simulink model "simcape_real_time_V3"  (R2022b)
settings: Solver=FixedStepAuto  StartTime=0.0  StopTime=100  FixedStep=0.002  RelTol=1e-3
undefined symbols (not defined in the file): drone_leg, K_LQR_GOC, pitch_init, roll_init, v_pitch_init, v_roll_init, v_x_init, v_y_init, v_yaw_init, v_z_init, X, x_init, Y, y_init, yaw_init, Z, z_init
libraries: sm_lib x70, nesl_utility x11, simulink x6
(part 3 of 4)

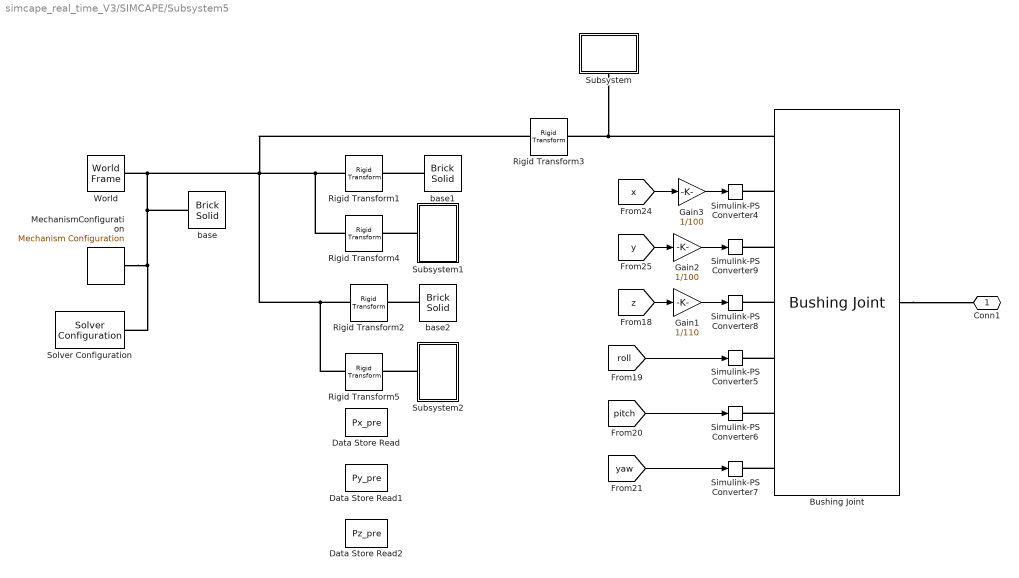
== system simcape_real_time_V3/SIMCAPE/Subsystem5 ==
  Bushing Joint : sm_lib/Joints/Bushing Joint  JointMode=Normal  SenseConstraintForce=off  SenseConstraintForceX=off  SenseConstraintForceY=off  SenseConstraintForceZ=off  SenseConstraintTorque=off  SenseConstraintTorqueX=off  SenseConstraintTorqueY=off  SenseConstraintTorqueZ=off  SenseTotalForce=off  SenseTotalForceX=off  SenseTotalForceY=off  SenseTotalForceZ=off  SenseTotalTorque=off  SenseTotalTorqueX=off  SenseTotalTorqueY=off  SenseTotalTorqueZ=off  CompositeWrenchDir=FollowerOnBase  CompositeWrenchFrame=BaseFrame  PxEquilibriumPosition=0  PxEquilibriumPositionUnits=m  PxSpringStiffness=0  PxSpringStiffnessUnits=N/m  PxDampingCoefficient=0  PxDampingCoefficientUnits=N/(m/s)  PxTorqueActuationMode=ComputedTorque  PxMotionActuationMode=InputMotion  PxSensePosition=off  PxSenseVelocity=off  PxSenseAcceleration=off  PxSenseTorqueForce=off  PxSenseLowerLimitTorqueForce=off  PxSenseUpperLimitTorqueForce=off  PxLowerLimitSpecify=off  PxLowerLimitBound=-1  PxLowerLimitBoundUnits=m  PxLowerLimitStiffness=1e6  PxLowerLimitStiffnessUnits=N/m  PxLowerLimitDamping=1e3  PxLowerLimitDampingUnits=N/(m/s)  PxLowerLimitTransitionRegionWidth=1e-4  PxLowerLimitTransitionRegionWidthUnits=m  PxUpperLimitSpecify=off  PxUpperLimitBound=1  PxUpperLimitBoundUnits=m  PxUpperLimitStiffness=1e6  PxUpperLimitStiffnessUnits=N/m  PxUpperLimitDamping=1e3  PxUpperLimitDampingUnits=N/(m/s)  PxUpperLimitTransitionRegionWidth=1e-4  PxUpperLimitTransitionRegionWidthUnits=m  PxPositionTargetSpecify=off  PxPositionTargetPriority=High  PxPositionTargetValue=0  PxPositionTargetValueUnits=m  PxVelocityTargetSpecify=off  PxVelocityTargetPriority=High  PxVelocityTargetValue=0  PxVelocityTargetValueUnits=m/s  PyEquilibriumPosition=0  PyEquilibriumPositionUnits=m  PySpringStiffness=0  PySpringStiffnessUnits=N/m  PyDampingCoefficient=0  PyDampingCoefficientUnits=N/(m/s)  PyTorqueActuationMode=ComputedTorque  PyMotionActuationMode=InputMotion  PySensePosition=off  PySenseVelocity=off  PySenseAcceleration=off  PySenseTorqueForce=off  PySenseLowerLimitTorqueForce=off  PySenseUpperLimitTorqueForce=off  PyLowerLimitSpecify=off  PyLowerLimitBound=-1  PyLowerLimitBoundUnits=m  PyLowerLimitStiffness=1e6  PyLowerLimitStiffnessUnits=N/m  PyLowerLimitDamping=1e3  PyLowerLimitDampingUnits=N/(m/s)  PyLowerLimitTransitionRegionWidth=1e-4  PyLowerLimitTransitionRegionWidthUnits=m  PyUpperLimitSpecify=off  PyUpperLimitBound=1  PyUpperLimitBoundUnits=m  PyUpperLimitStiffness=1e6  PyUpperLimitStiffnessUnits=N/m  PyUpperLimitDamping=1e3  PyUpperLimitDampingUnits=N/(m/s)  PyUpperLimitTransitionRegionWidth=1e-4  PyUpperLimitTransitionRegionWidthUnits=m  PyPositionTargetSpecify=off  PyPositionTargetPriority=High  PyPositionTargetValue=0  PyPositionTargetValueUnits=m  PyVelocityTargetSpecify=off  PyVelocityTargetPriority=High  PyVelocityTargetValue=0  PyVelocityTargetValueUnits=m/s  PzEquilibriumPosition=0  PzEquilibriumPositionUnits=m  PzSpringStiffness=0  PzSpringStiffnessUnits=N/m  PzDampingCoefficient=0  PzDampingCoefficientUnits=N/(m/s)  PzTorqueActuationMode=ComputedTorque  PzMotionActuationMode=InputMotion  PzSensePosition=off  PzSenseVelocity=off  PzSenseAcceleration=off  PzSenseTorqueForce=off  PzSenseLowerLimitTorqueForce=off  PzSenseUpperLimitTorqueForce=off  PzLowerLimitSpecify=off  PzLowerLimitBound=-1  PzLowerLimitBoundUnits=m  PzLowerLimitStiffness=1e6  PzLowerLimitStiffnessUnits=N/m  PzLowerLimitDamping=1e3  PzLowerLimitDampingUnits=N/(m/s)  PzLowerLimitTransitionRegionWidth=1e-4  PzLowerLimitTransitionRegionWidthUnits=m  PzUpperLimitSpecify=off  PzUpperLimitBound=1  PzUpperLimitBoundUnits=m  PzUpperLimitStiffness=1e6  PzUpperLimitStiffnessUnits=N/m  PzUpperLimitDamping=1e3  PzUpperLimitDampingUnits=N/(m/s)  PzUpperLimitTransitionRegionWidth=1e-4  PzUpperLimitTransitionRegionWidthUnits=m  PzPositionTargetSpecify=off  PzPositionTargetPriority=High  PzPositionTargetValue=0  PzPositionTargetValueUnits=m  PzVelocityTargetSpecify=off  PzVelocityTargetPriority=High  PzVelocityTargetValue=0  PzVelocityTargetValueUnits=m/s  RxEquilibriumPosition=0  RxEquilibriumPositionUnits=deg  RxSpringStiffness=0  RxSpringStiffnessUnits=N*m/deg  RxDampingCoefficient=0  RxDampingCoefficientUnits=N*m/(deg/s)  RxTorqueActuationMode=ComputedTorque  RxMotionActuationMode=InputMotion  RxSensePosition=off  RxSenseVelocity=off  RxSenseAcceleration=off  RxSenseTorqueForce=off  RxSenseLowerLimitTorqueForce=off  RxSenseUpperLimitTorqueForce=off  RxLowerLimitSpecify=off  RxLowerLimitBound=-90  RxLowerLimitBoundUnits=deg  RxLowerLimitStiffness=1e4  RxLowerLimitStiffnessUnits=N*m/deg  RxLowerLimitDamping=10  RxLowerLimitDampingUnits=N*m/(deg/s)  RxLowerLimitTransitionRegionWidth=0.1  RxLowerLimitTransitionRegionWidthUnits=deg  RxUpperLimitSpecify=off  RxUpperLimitBound=90  RxUpperLimitBoundUnits=deg  RxUpperLimitStiffness=1e4  RxUpperLimitStiffnessUnits=N*m/deg  RxUpperLimitDamping=10  RxUpperLimitDampingUnits=N*m/(deg/s)  RxUpperLimitTransitionRegionWidth=0.1  RxUpperLimitTransitionRegionWidthUnits=deg  RxPositionTargetSpecify=off  RxPositionTargetPriority=High  RxPositionTargetValue=0  RxPositionTargetValueUnits=deg  RxVelocityTargetSpecify=off  RxVelocityTargetPriority=High  RxVelocityTargetValue=0  RxVelocityTargetValueUnits=deg/s  RyEquilibriumPosition=0  RyEquilibriumPositionUnits=deg  RySpringStiffness=0  RySpringStiffnessUnits=N*m/deg  RyDampingCoefficient=0  RyDampingCoefficientUnits=N*m/(deg/s)  RyTorqueActuationMode=ComputedTorque  RyMotionActuationMode=InputMotion  RySensePosition=off  RySenseVelocity=off  RySenseAcceleration=off  RySenseTorqueForce=off  RySenseLowerLimitTorqueForce=off  RySenseUpperLimitTorqueForce=off  RyLowerLimitSpecify=off  RyLowerLimitBound=-90  RyLowerLimitBoundUnits=deg  RyLowerLimitStiffness=1e4  RyLowerLimitStiffnessUnits=N*m/deg  RyLowerLimitDamping=10  RyLowerLimitDampingUnits=N*m/(deg/s)  RyLowerLimitTransitionRegionWidth=0.1  RyLowerLimitTransitionRegionWidthUnits=deg  RyUpperLimitSpecify=off  RyUpperLimitBound=90  RyUpperLimitBoundUnits=deg  RyUpperLimitStiffness=1e4  RyUpperLimitStiffnessUnits=N*m/deg  RyUpperLimitDamping=10  RyUpperLimitDampingUnits=N*m/(deg/s)  RyUpperLimitTransitionRegionWidth=0.1  RyUpperLimitTransitionRegionWidthUnits=deg  RyPositionTargetSpecify=off  RyPositionTargetPriority=High  RyPositionTargetValue=0  RyPositionTargetValueUnits=deg  RyVelocityTargetSpecify=off  RyVelocityTargetPriority=High  RyVelocityTargetValue=0  RyVelocityTargetValueUnits=deg/s  RzEquilibriumPosition=0  RzEquilibriumPositionUnits=deg  RzSpringStiffness=0  RzSpringStiffnessUnits=N*m/deg  RzDampingCoefficient=0  RzDampingCoefficientUnits=N*m/(deg/s)  RzTorqueActuationMode=ComputedTorque  RzMotionActuationMode=InputMotion  RzSensePosition=off  RzSenseVelocity=off  RzSenseAcceleration=off  RzSenseTorqueForce=off  RzSenseLowerLimitTorqueForce=off  RzSenseUpperLimitTorqueForce=off  RzLowerLimitSpecify=off  RzLowerLimitBound=-90  RzLowerLimitBoundUnits=deg  RzLowerLimitStiffness=1e4  RzLowerLimitStiffnessUnits=N*m/deg  RzLowerLimitDamping=10  RzLowerLimitDampingUnits=N*m/(deg/s)  RzLowerLimitTransitionRegionWidth=0.1  RzLowerLimitTransitionRegionWidthUnits=deg  RzUpperLimitSpecify=off  RzUpperLimitBound=90  RzUpperLimitBoundUnits=deg  RzUpperLimitStiffness=1e4  RzUpperLimitStiffnessUnits=N*m/deg  RzUpperLimitDamping=10  RzUpperLimitDampingUnits=N*m/(deg/s)  RzUpperLimitTransitionRegionWidth=0.1  RzUpperLimitTransitionRegionWidthUnits=deg  RzPositionTargetSpecify=off  RzPositionTargetPriority=High  RzPositionTargetValue=0  RzPositionTargetValueUnits=deg  RzVelocityTargetSpecify=off  RzVelocityTargetPriority=High  RzVelocityTargetValue=0  RzVelocityTargetValueUnits=deg/s
  Data Store Read : DataStoreRead  DataStoreName=Px_pre  IndexOptions=Index vector (dialog)  Indices=1  OutputSizes=1
  Data Store Read1 : DataStoreRead  DataStoreName=Py_pre  IndexOptions=Index vector (dialog)  Indices=1  OutputSizes=1
  Data Store Read2 : DataStoreRead  DataStoreName=Pz_pre  IndexOptions=Index vector (dialog)  Indices=1  OutputSizes=1
  Gain1 : Gain  Gain=1/110
  Gain2 : Gain  Gain=1/100
  Gain3 : Gain  Gain=1/100
  MechanismConfiguration : sm_lib/Utilities/Mechanism Configuration  UniformGravity=Constant  GravityVector=[0 -9.81 0]  GravityUnits=m/s^2  LinearizationDelta=0.002  JointModeTransitionNonlinearIterations=2
  Rigid Transform1 : sm_lib/Frames and Transforms/Rigid Transform  TranslationMethod=Cartesian  TranslationStandardOffset=45  TranslationLengthUnit=cm  TranslationStandardAxis=+Y  TranslationCartesianOffset=[0 300 -50]  TranslationROffset=0  TranslationROffsetUnits=m  TranslationZOffset=0  TranslationZOffsetUnits=m  TranslationThetaOffset=0  TranslationThetaOffsetUnits=deg  RotationMethod=StandardAxis  RotationAngleUnits=deg  RotationStandardAxis=+Z  RotationAngle=90  RotationArbitraryAxis=[0 0 1]  FollAlignAxisA=+X  BaseAlignAxisA=+Y  FollAlignAxisB=+Y  BaseAlignAxisB=+Z  RotationSequenceAxes=FollowerAxes  RotationSequence=XYX  RotationSequenceAngles=[0 0 0]  RotationSequenceAnglesUnits=deg  RotationMatrix=[1 0 0; 0 1 0; 0 0 1]  Quaternion=[1 0 0 0]
  Rigid Transform2 : sm_lib/Frames and Transforms/Rigid Transform  TranslationMethod=Cartesian  TranslationStandardOffset=45  TranslationLengthUnit=cm  TranslationStandardAxis=+Y  TranslationCartesianOffset=[300 0 -100]  TranslationROffset=0  TranslationROffsetUnits=m  TranslationZOffset=0  TranslationZOffsetUnits=m  TranslationThetaOffset=0  TranslationThetaOffsetUnits=deg  RotationMethod=StandardAxis  RotationAngleUnits=deg  RotationStandardAxis=+Z  RotationAngle=90  RotationArbitraryAxis=[0 0 1]  FollAlignAxisA=+X  BaseAlignAxisA=+Y  FollAlignAxisB=+Y  BaseAlignAxisB=+Z  RotationSequenceAxes=FollowerAxes  RotationSequence=XYX  RotationSequenceAngles=[0 0 0]  RotationSequenceAnglesUnits=deg  RotationMatrix=[1 0 0; 0 1 0; 0 0 1]  Quaternion=[1 0 0 0]
  Rigid Transform3 : sm_lib/Frames and Transforms/Rigid Transform  TranslationMethod=Cartesian  TranslationStandardOffset=45  TranslationLengthUnit=cm  TranslationStandardAxis=+Y  TranslationCartesianOffset=[0 -0 -30]  TranslationROffset=0  TranslationROffsetUnits=m  TranslationZOffset=0  TranslationZOffsetUnits=m  TranslationThetaOffset=0  TranslationThetaOffsetUnits=deg  RotationMethod=StandardAxis  RotationAngleUnits=deg  RotationStandardAxis=+Z  RotationAngle=90  RotationArbitraryAxis=[0 0 1]  FollAlignAxisA=+X  BaseAlignAxisA=+Y  FollAlignAxisB=+Y  BaseAlignAxisB=+Z  RotationSequenceAxes=FollowerAxes  RotationSequence=XYX  RotationSequenceAngles=[0 0 0]  RotationSequenceAnglesUnits=deg  RotationMatrix=[1 0 0; 0 1 0; 0 0 1]  Quaternion=[1 0 0 0]
  Rigid Transform4 : sm_lib/Frames and Transforms/Rigid Transform  TranslationMethod=Cartesian  TranslationStandardOffset=45  TranslationLengthUnit=cm  TranslationStandardAxis=+Y  TranslationCartesianOffset=[0 300 -80]  TranslationROffset=0  TranslationROffsetUnits=m  TranslationZOffset=0  TranslationZOffsetUnits=m  TranslationThetaOffset=0  TranslationThetaOffsetUnits=deg  RotationMethod=StandardAxis  RotationAngleUnits=deg  RotationStandardAxis=+Z  RotationAngle=90  RotationArbitraryAxis=[0 0 1]  FollAlignAxisA=+X  BaseAlignAxisA=+Y  FollAlignAxisB=+Y  BaseAlignAxisB=+Z  RotationSequenceAxes=FollowerAxes  RotationSequence=XYX  RotationSequenceAngles=[0 0 0]  RotationSequenceAnglesUnits=deg  RotationMatrix=[1 0 0; 0 1 0; 0 0 1]  Quaternion=[1 0 0 0]
  Rigid Transform5 : sm_lib/Frames and Transforms/Rigid Transform  TranslationMethod=Cartesian  TranslationStandardOffset=45  TranslationLengthUnit=cm  TranslationStandardAxis=+Y  TranslationCartesianOffset=[300 0 -130]  TranslationROffset=0  TranslationROffsetUnits=m  TranslationZOffset=0  TranslationZOffsetUnits=m  TranslationThetaOffset=0  TranslationThetaOffsetUnits=deg  RotationMethod=StandardAxis  RotationAngleUnits=deg  RotationStandardAxis=+Z  RotationAngle=90  RotationArbitraryAxis=[0 0 1]  FollAlignAxisA=+X  BaseAlignAxisA=+Y  FollAlignAxisB=+Y  BaseAlignAxisB=+Z  RotationSequenceAxes=FollowerAxes  RotationSequence=XYX  RotationSequenceAngles=[0 0 0]  RotationSequenceAnglesUnits=deg  RotationMatrix=[1 0 0; 0 1 0; 0 0 1]  Quaternion=[1 0 0 0]
  Simulink-PS Converter{4..9} (6 alike) : nesl_utility/Simulink-PS Converter  PhysicalDomain=network_engine_domain  SubClassName=ps_input  LeftPortType=input  RightPortType=output  PseudoPeriodic=off  Frequencies=[]  NoiseDistribution=none  NoiseParameters=[]  Unit=1  AffineConversion=off  FilteringAndDerivatives=filter  SimscapeFilterOrder=2  InputFilterTimeConstant=0.002  UdotUserProvided=0
  Solver Configuration : nesl_utility/Solver Configuration  PhysicalDomain=network_engine_domain  SubClassName=solver  LeftPortType=input  RightPortType=generic  Tones=[]  Harmonics=[]  SimulateNoise=off  Profile=off  UseLocalSampling=off  EnableSwitchedLinearOptims=on  FrequencyDomain=off  UseCCode=off  RelTol=0.001  AbsTol=1e-06  MinStep=1e-09  ToWorkspace=off  RevertToSquareIcSolve=off  NumHomotopyIterations=100  PhasorMode=off  PhasorModeNumHarmonics=1  ConsistencySolver=NEWTON_FTOL  IndexReductionMethod=DerivativeReplacement  DoDC=off  ResidualTolerance=1e-09  ConsistencyTolSource=GLOBAL  ConsistencyAbsTol=0.001  ConsistencyRelTol=0.001  ConsistencyTolFactor=0.001  UseLocalSolver=off  LocalSolverChoice=NE_BACKWARD_EULER_ADVANCER  ResolveIndetEquations=on  FunctionEvalNumThread=1  LocalSolverSampleTime=0.001  DoFixedCost=off  MaxNonlinIter=3  MaxModeIter=2  ComputeImpulses=off  ImpulseIterations=2  LinearAlgebra=Sparse  LinearAlgebraNumThread=0  EquationFormulation=NE_TIME_EF  DelaysMemoryBudget=1024  AutomaticFiltering=on  FilteringTimeConstant=0.001  PartitionStorageMethod=AS_NEEDED  PartitionMemoryBudget=1024  PartitionMethod=FAST
  Subsystem : Subsystem
  Subsystem1 : Subsystem
  Subsystem2 : Subsystem
  World : sm_lib/Frames and Transforms/World Frame
  base : sm_lib/Body Elements/Brick Solid  GraphicAmbientColor=[0.15 0.9 0.15 1.0]  BasedOnType=Density  BrickDimensions=[300 300 50]  BrickDimensionUnits=cm  CenterOfMass=[0 0 0]  CenterOfMassUnits=m  GraphicDiffuseColor=[0.0 0.8 0.0]  Density=1000  DensityUnits=kg/(m^3)  DoExposeReferenceFrame=on  GraphicEmissiveColor=[0.0 0.0 0.0 1.0]  ExportEntireGeometry=off  SerializedFrames=<Frames/>  MarkerShape=Sphere  MarkerSize=10  GraphicType=FromGeometry  InertiaType=CalculateFromGeometry  Mass=1  MassUnits=kg  MomentsOfInertia=[1 1 1]  MomentsOfInertiaUnits=kg*m^2  GraphicOpacity=1.0  ProductsOfInertia=[0 0 0]  ProductsOfInertiaUnits=kg*m^2  GraphicShininess=75  GraphicSpecularColor=[0.5 0.5 0.5 1.0]  GraphicVisPropType=SimpleVisualProperties
  base1 : sm_lib/Body Elements/Brick Solid  GraphicAmbientColor=[0.15 0.9 0.15 1.0]  BasedOnType=Density  BrickDimensions=[300 300 50]  BrickDimensionUnits=cm  CenterOfMass=[0 0 0]  CenterOfMassUnits=m  GraphicDiffuseColor=[0.4 1.0 1.0]  Density=1000  DensityUnits=kg/(m^3)  DoExposeReferenceFrame=on  GraphicEmissiveColor=[0.0 0.0 0.0 1.0]  ExportEntireGeometry=off  SerializedFrames=<Frames/>  MarkerShape=Sphere  MarkerSize=10  GraphicType=FromGeometry  InertiaType=CalculateFromGeometry  Mass=1  MassUnits=kg  MomentsOfInertia=[1 1 1]  MomentsOfInertiaUnits=kg*m^2  GraphicOpacity=1.0  ProductsOfInertia=[0 0 0]  ProductsOfInertiaUnits=kg*m^2  GraphicShininess=75  GraphicSpecularColor=[0.5 0.5 0.5 1.0]  GraphicVisPropType=SimpleVisualProperties
  base2 : sm_lib/Body Elements/Brick Solid  GraphicAmbientColor=[0.15 0.9 0.15 1.0]  BasedOnType=Density  BrickDimensions=[300 300 50]  BrickDimensionUnits=cm  CenterOfMass=[0 0 0]  CenterOfMassUnits=m  GraphicDiffuseColor=[1.0 1.0 0.8]  Density=1000  DensityUnits=kg/(m^3)  DoExposeReferenceFrame=on  GraphicEmissiveColor=[0.0 0.0 0.0 1.0]  ExportEntireGeometry=off  SerializedFrames=<Frames/>  MarkerShape=Sphere  MarkerSize=10  GraphicType=FromGeometry  InertiaType=CalculateFromGeometry  Mass=1  MassUnits=kg  MomentsOfInertia=[1 1 1]  MomentsOfInertiaUnits=kg*m^2  GraphicOpacity=1.0  ProductsOfInertia=[0 0 0]  ProductsOfInertiaUnits=kg*m^2  GraphicShininess=75  GraphicSpecularColor=[0.5 0.5 0.5 1.0]  GraphicVisPropType=SimpleVisualProperties
  Conn1 : PMIOPort  Side=Right
  wires:
  [pitch] -> Simulink-PS Converter6/1
  [roll] -> Simulink-PS Converter5/1
  Gain3/1 -> Simulink-PS Converter4/1
  Gain1/1 -> Simulink-PS Converter8/1
  Gain2/1 -> Simulink-PS Converter9/1
  [yaw] -> Simulink-PS Converter7/1
  [x] -> Gain3/1
  [y] -> Gain2/1
  [z] -> Gain1/1
  connections:
  base/RConn1 -- MechanismConfiguration/RConn1 -- Solver Configuration/RConn1 -- Rigid Transform5/RConn1 -- Rigid Transform2/RConn1 -- Rigid Transform4/RConn1 -- Rigid Transform1/RConn1 -- Rigid Transform3/RConn1 -- World/RConn1
  Bushing Joint/LConn4 -- Simulink-PS Converter8/RConn1
  Bushing Joint/LConn6 -- Simulink-PS Converter6/RConn1
  Bushing Joint/LConn1 -- Subsystem/LConn1 -- Rigid Transform3/LConn1
  Bushing Joint/LConn5 -- Simulink-PS Converter5/RConn1
  Bushing Joint/LConn7 -- Simulink-PS Converter7/RConn1
  Bushing Joint/LConn3 -- Simulink-PS Converter9/RConn1
  Bushing Joint/LConn2 -- Simulink-PS Converter4/RConn1
  Bushing Joint/RConn1 -- Conn1/RConn1
  base1/RConn1 -- Rigid Transform1/LConn1
  base2/RConn1 -- Rigid Transform2/LConn1
  Subsystem1/LConn1 -- Rigid Transform4/LConn1
  Subsystem2/LConn1 -- Rigid Transform5/LConn1

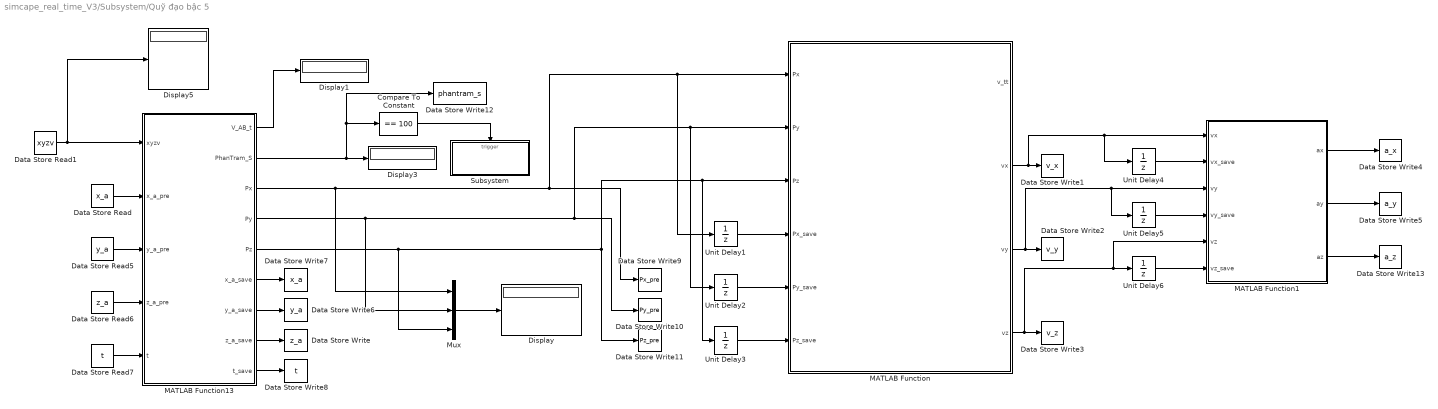
== system simcape_real_time_V3/Subsystem/Quỹ đạo bậc 5 ==
  Compare To Constant : simulink/Logic and Bit Operations/Compare To Constant  relop===  const=100  OutDataTypeStr=boolean
  Data Store Read : DataStoreRead  DataStoreName=x_a  IndexOptions=Index vector (dialog)  Indices=1  OutputSizes=1
  Data Store Read1 : DataStoreRead  DataStoreName=xyzv  IndexOptions=Index vector (dialog)  Indices=1  OutputSizes=1
  Data Store Read5 : DataStoreRead  DataStoreName=y_a  IndexOptions=Index vector (dialog)  Indices=1  OutputSizes=1
  Data Store Read6 : DataStoreRead  DataStoreName=z_a  IndexOptions=Index vector (dialog)  Indices=1  OutputSizes=1
  Data Store Read7 : DataStoreRead  DataStoreName=t  IndexOptions=Index vector (dialog)  Indices=1  OutputSizes=1
  Data Store Write : DataStoreWrite  DataStoreName=z_a  IndexOptions=Index vector (dialog)  Indices=1  OutputSizes=1
  Data Store Write1 : DataStoreWrite  DataStoreName=v_x  IndexOptions=Index vector (dialog)  Indices=1  OutputSizes=1
  Data Store Write10 : DataStoreWrite  DataStoreName=Py_pre  IndexOptions=Index vector (dialog)  Indices=1  OutputSizes=1
  Data Store Write11 : DataStoreWrite  DataStoreName=Pz_pre  IndexOptions=Index vector (dialog)  Indices=1  OutputSizes=1
  Data Store Write12 : DataStoreWrite  DataStoreName=phantram_s  DataStoreElements=phantram_s  IndexOptions=Index vector (dialog)  Indices=1  OutputSizes=1
  Data Store Write13 : DataStoreWrite  DataStoreName=a_z  IndexOptions=Index vector (dialog)  Indices=1  OutputSizes=1
  Data Store Write2 : DataStoreWrite  DataStoreName=v_y  IndexOptions=Index vector (dialog)  Indices=1  OutputSizes=1
  Data Store Write3 : DataStoreWrite  DataStoreName=v_z  IndexOptions=Index vector (dialog)  Indices=1  OutputSizes=1
  Data Store Write4 : DataStoreWrite  DataStoreName=a_x  IndexOptions=Index vector (dialog)  Indices=1  OutputSizes=1
  Data Store Write5 : DataStoreWrite  DataStoreName=a_y  IndexOptions=Index vector (dialog)  Indices=1  OutputSizes=1
  Data Store Write6 : DataStoreWrite  DataStoreName=y_a  IndexOptions=Index vector (dialog)  Indices=1  OutputSizes=1
  Data Store Write7 : DataStoreWrite  DataStoreName=x_a  IndexOptions=Index vector (dialog)  Indices=1  OutputSizes=1
  Data Store Write8 : DataStoreWrite  DataStoreName=t  IndexOptions=Index vector (dialog)  Indices=1  OutputSizes=1
  Data Store Write9 : DataStoreWrite  DataStoreName=Px_pre  IndexOptions=Index vector (dialog)  Indices=1  OutputSizes=1
  Display{,1,3,5} (4 alike) : Display
  MATLAB Function : MATLAB Function  TreatAsAtomicUnit=on
  MATLAB Function1 : MATLAB Function  TreatAsAtomicUnit=on
  MATLAB Function13 : MATLAB Function  TreatAsAtomicUnit=on
  Mux : Mux  Inputs=3
  Subsystem : Subsystem
  Unit Delay{1..6} (6 alike) : UnitDelay  SampleTime=-1  HasFrameUpgradeWarning=on
  wires:
  MATLAB Function13/9(t_save) -> Data Store Write8/1
  Compare To Constant/1 -> Subsystem/Trigger
  MATLAB Function13/2(PhanTram_S) -> Data Store Write12/1, Compare To Constant/1, Display3/1
  Data Store Read/1 -> MATLAB Function13/2(x_a_pre)
  Data Store Read6/1 -> MATLAB Function13/4(z_a_pre)
  MATLAB Function13/8(z_a_save) -> Data Store Write/1
  Data Store Read1/1 -> Display5/1, MATLAB Function13/1(xyzv)
  MATLAB Function13/6(x_a_save) -> Data Store Write7/1
  MATLAB Function13/7(y_a_save) -> Data Store Write6/1
  Data Store Read7/1 -> MATLAB Function13/5(t)
  Data Store Read5/1 -> MATLAB Function13/3(y_a_pre)
  Unit Delay4/1 -> MATLAB Function1/2(vx_save)
  MATLAB Function13/4(Py) -> Mux/2, Unit Delay2/1, MATLAB Function/2(Py), Data Store Write10/1
  Unit Delay2/1 -> MATLAB Function/5(Py_save)
  Unit Delay1/1 -> MATLAB Function/4(Px_save)
  Unit Delay3/1 -> MATLAB Function/6(Pz_save)
  Mux/1 -> Display/1
  MATLAB Function/4(vz) -> Unit Delay6/1, MATLAB Function1/5(vz), Data Store Write3/1
  MATLAB Function/3(vy) -> Unit Delay5/1, MATLAB Function1/3(vy), Data Store Write2/1
  MATLAB Function/2(vx) -> Unit Delay4/1, MATLAB Function1/1(vx), Data Store Write1/1
  MATLAB Function1/1(ax) -> Data Store Write4/1
  MATLAB Function1/2(ay) -> Data Store Write5/1
  MATLAB Function1/3(az) -> Data Store Write13/1
  Unit Delay5/1 -> MATLAB Function1/4(vy_save)
  Unit Delay6/1 -> MATLAB Function1/6(vz_save)
  MATLAB Function13/3(Px) -> Mux/1, Unit Delay1/1, MATLAB Function/1(Px), Data Store Write9/1
  MATLAB Function13/5(Pz) -> Mux/3, Unit Delay3/1, MATLAB Function/3(Pz), Data Store Write11/1
  MATLAB Function13/1(V_AB_t) -> Display1/1

== system simcape_real_time_V3/Subsystem1/Quỹ đạo trục x ==
  qf_x : Inport
  v_qd_x : Inport  Port=2
  Constant40 : Constant  Value=0
  MATLAB Function10 : MATLAB Function  TreatAsAtomicUnit=on
  X_x : Outport
  V_x : Outport  Port=2
  A_x : Outport  Port=3
  tag scope: A_x=global, V_x=global, X_x=global
  wires:
  Constant40/1 -> MATLAB Function10/1(q0)
  v_qd_x/1 -> MATLAB Function10/3(v_qd)
  qf_x/1 -> MATLAB Function10/2(qf)
  MATLAB Function10/1(X) -> [X_x], X_x/1
  MATLAB Function10/3(A) -> [A_x], A_x/1
  MATLAB Function10/2(V) -> [V_x], V_x/1

== system simcape_real_time_V3/Subsystem1/Quỹ đạo trục y ==
  qf_y : Inport
  v_qd_y : Inport  Port=2
  Constant40 : Constant  Value=0
  MATLAB Function10 : MATLAB Function  TreatAsAtomicUnit=on
  X_y : Outport
  V_y : Outport  Port=2
  A_y : Outport  Port=3
  tag scope: A_y=global, V_y=global, X_y=global
  wires:
  Constant40/1 -> MATLAB Function10/1(q0)
  v_qd_y/1 -> MATLAB Function10/3(v_qd)
  qf_y/1 -> MATLAB Function10/2(qf)
  MATLAB Function10/1(X) -> [X_y], X_y/1
  MATLAB Function10/2(V) -> [V_y], V_y/1
  MATLAB Function10/3(A) -> A_y/1, [A_y]

== system simcape_real_time_V3/Subsystem1/Quỹ đạo trục z ==
  qf_z : Inport
  v_qd_z : Inport  Port=2
  Constant40 : Constant  Value=0
  MATLAB Function10 : MATLAB Function  TreatAsAtomicUnit=on
  X_z : Outport
  V_z : Outport  Port=2
  A_z : Outport  Port=3
  tag scope: A_z=global, V_z=global, X_z=global
  wires:
  Constant40/1 -> MATLAB Function10/1(q0)
  v_qd_z/1 -> MATLAB Function10/3(v_qd)
  qf_z/1 -> MATLAB Function10/2(qf)
  MATLAB Function10/2(V) -> [V_z], V_z/1
  MATLAB Function10/3(A) -> [A_z], A_z/1
  MATLAB Function10/1(X) -> [X_z], X_z/1

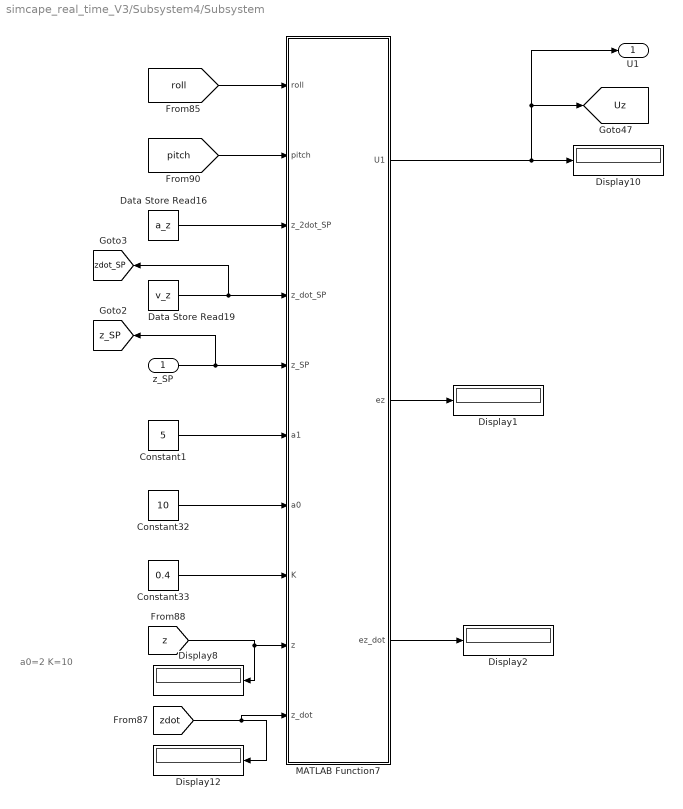
== system simcape_real_time_V3/Subsystem4/Subsystem ==
  note: a0=2
      | K=10
  z_SP : Inport
  Constant1 : Constant  Value=5
  Constant32 : Constant  Value=10
  Constant33 : Constant  Value=0.4
  Data Store Read16 : DataStoreRead  DataStoreName=a_z  IndexOptions=Index vector (dialog)  Indices=1  OutputSizes=1
  Data Store Read19 : DataStoreRead  DataStoreName=v_z  IndexOptions=Index vector (dialog)  Indices=1  OutputSizes=1
  Display{1..2,8,10,12} (5 alike) : Display
  MATLAB Function7 : MATLAB Function  TreatAsAtomicUnit=on
  U1 : Outport
  tag scope: Uz=global, z_SP=global, zdot_SP=global
  wires:
  [z] -> Display8/1, MATLAB Function7/9(z)
  Constant32/1 -> MATLAB Function7/7(a0)
  [zdot] -> Display12/1, MATLAB Function7/10(z_dot)
  [pitch] -> MATLAB Function7/2(pitch)
  Constant33/1 -> MATLAB Function7/8(K)
  [roll] -> MATLAB Function7/1(roll)
  MATLAB Function7/1(U1) -> U1/1, [Uz], Display10/1
  MATLAB Function7/2(ez) -> Display1/1
  MATLAB Function7/3(ez_dot) -> Display2/1
  z_SP/1 -> [z_SP], MATLAB Function7/5(z_SP)
  Data Store Read16/1 -> MATLAB Function7/3(z_2dot_SP)
  Data Store Read19/1 -> [zdot_SP], MATLAB Function7/4(z_dot_SP)
  Constant1/1 -> MATLAB Function7/6(a1)

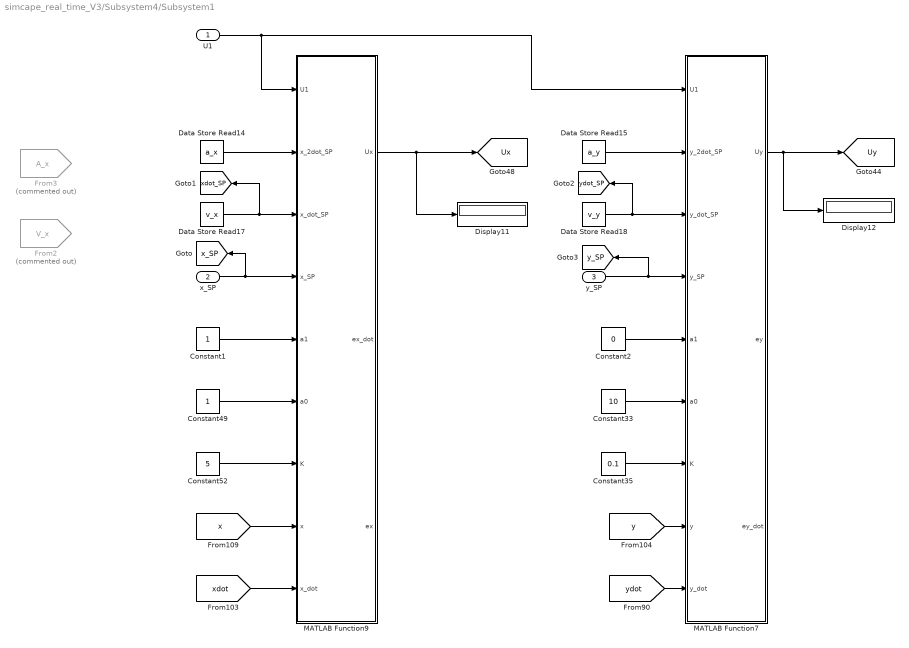
== system simcape_real_time_V3/Subsystem4/Subsystem1 ==
  U1 : Inport
  x_SP : Inport  Port=2
  y_SP : Inport  Port=3
  Constant1 : Constant
  Constant2 : Constant  Value=0
  Constant33 : Constant  Value=10
  Constant35 : Constant  Value=0.1
  Constant49 : Constant
  Constant52 : Constant  Value=5
  Data Store Read14 : DataStoreRead  DataStoreName=a_x  IndexOptions=Index vector (dialog)  Indices=1  OutputSizes=1
  Data Store Read15 : DataStoreRead  DataStoreName=a_y  IndexOptions=Index vector (dialog)  Indices=1  OutputSizes=1
  Data Store Read17 : DataStoreRead  DataStoreName=v_x  IndexOptions=Index vector (dialog)  Indices=1  OutputSizes=1
  Data Store Read18 : DataStoreRead  DataStoreName=v_y  IndexOptions=Index vector (dialog)  Indices=1  OutputSizes=1
  Display11 : Display
  Display12 : Display
  From2 : From  Commented=on  GotoTag=V_x  TagVisibility=global
  From3 : From  Commented=on  GotoTag=A_x  TagVisibility=global
  MATLAB Function7 : MATLAB Function  TreatAsAtomicUnit=on
  MATLAB Function9 : MATLAB Function  TreatAsAtomicUnit=on
  tag scope: Ux=global, Uy=global, x_SP=global, xdot_SP=global, y_SP=global, ydot_SP=global
  wires:
  Constant49/1 -> MATLAB Function9/6(a0)
  [x] -> MATLAB Function9/8(x)
  Constant52/1 -> MATLAB Function9/7(K)
  [xdot] -> MATLAB Function9/9(x_dot)
  x_SP/1 -> [x_SP], MATLAB Function9/4(x_SP)
  MATLAB Function9/1(Ux) -> Display11/1, [Ux]
  y_SP/1 -> [y_SP], MATLAB Function7/4(y_SP)
  U1/1 -> MATLAB Function7/1(U1), MATLAB Function9/1(U1)
  [ydot] -> MATLAB Function7/9(y_dot)
  Constant33/1 -> MATLAB Function7/6(a0)
  Constant35/1 -> MATLAB Function7/7(K)
  MATLAB Function7/1(Uy) -> Display12/1, [Uy]
  [y] -> MATLAB Function7/8(y)
  Data Store Read17/1 -> [xdot_SP], MATLAB Function9/3(x_dot_SP)
  Data Store Read14/1 -> MATLAB Function9/2(x_2dot_SP)
  Data Store Read15/1 -> MATLAB Function7/2(y_2dot_SP)
  Data Store Read18/1 -> [ydot_SP], MATLAB Function7/3(y_dot_SP)
  Constant1/1 -> MATLAB Function9/5(a1)
  Constant2/1 -> MATLAB Function7/5(a1)

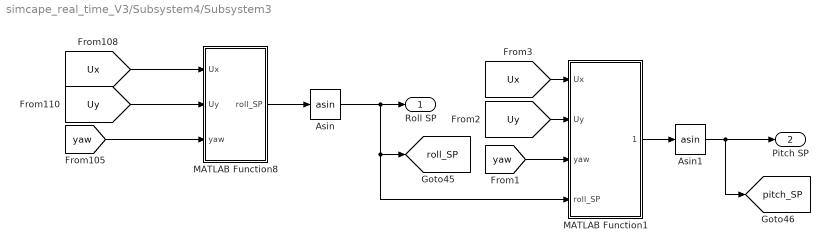
== system simcape_real_time_V3/Subsystem4/Subsystem3 ==
  Asin : Trigonometry  Operator=asin
  Asin1 : Trigonometry  Operator=asin
  MATLAB Function1 : MATLAB Function  TreatAsAtomicUnit=on
  MATLAB Function8 : MATLAB Function  TreatAsAtomicUnit=on
  Roll SP : Outport
  Pitch SP : Outport  Port=2
  tag scope: pitch_SP=global, roll_SP=global
  wires:
  [Ux] -> MATLAB Function8/1(Ux)
  [Uy] -> MATLAB Function8/2(Uy)
  MATLAB Function8/1(roll_SP) -> Asin/1
  Asin/1 -> Roll SP/1, MATLAB Function1/4(roll_SP), [roll_SP]
  [yaw] -> MATLAB Function8/3(yaw)
  [yaw] -> MATLAB Function1/3(yaw)
  [Uy] -> MATLAB Function1/2(Uy)
  [Ux] -> MATLAB Function1/1(Ux)
  Asin1/1 -> [pitch_SP], Pitch SP/1
  MATLAB Function1/1(pitch_SP) -> Asin1/1

== system simcape_real_time_V3/Nút Start/START/Subsystem ==
  Enable : EnablePort
  Constant1 : Constant
  Data Store Write1 : DataStoreWrite  DataStoreName=N_wp  DataStoreElements=N_wp  IndexOptions=Index vector (dialog)  Indices=1  OutputSizes=1
  wires:
  Constant1/1 -> Data Store Write1/1

== system simcape_real_time_V3/SIMCAPE/Subsystem5/Subsystem ==
  Target Inner Ring : sm_lib/Body Elements/Revolved Solid  GraphicAmbientColor=[0.15 0.15 0.15 1.0]  BasedOnType=Density  CenterOfMass=[0 0 0]  CenterOfMassUnits=m  GraphicDiffuseColor=[1.0 0.2 0.2]  ExportConvexHullGeometry=off  Density=1000  DensityUnits=kg/m^3  DoExposeReferenceFrame=on  GraphicEmissiveColor=[0.0 0.0 0.0 1.0]  ExportEntireGeometry=off  SerializedFrames=<Frames/>  MarkerShape=Sphere  MarkerSize=10  GraphicType=FromGeometry  InertiaType=CalculateFromGeometry  Mass=1  MassUnits=kg  MomentsOfInertia=[1 1 1]  MomentsOfInertiaUnits=kg*m^2  GraphicOpacity=1.0  ProductsOfInertia=[0 0 0]  ProductsOfInertiaUnits=kg*m^2  RevolutionCrossSection=[0.5 0.001; 0.5 -0.001; 0.75 -0.001; 0.75 0.001]*0.25  RevolutionCrossSectionUnits=m  RevolutionAngle=180  RevolutionAngleUnits=deg  RevolutionExtent=Full  GraphicShininess=75  GraphicSpecularColor=[0.5 0.5 0.5 1.0]  GraphicVisPropType=SimpleVisualProperties
  Target Middle Ring : sm_lib/Body Elements/Revolved Solid  GraphicAmbientColor=[0.15 0.15 0.15 1.0]  BasedOnType=Density  CenterOfMass=[0 0 0]  CenterOfMassUnits=m  GraphicDiffuseColor=[1.0 0.8 0.2]  ExportConvexHullGeometry=off  Density=1000  DensityUnits=kg/m^3  DoExposeReferenceFrame=on  GraphicEmissiveColor=[0.0 0.0 0.0 1.0]  ExportEntireGeometry=off  SerializedFrames=<Frames/>  MarkerShape=Sphere  MarkerSize=10  GraphicType=FromGeometry  InertiaType=CalculateFromGeometry  Mass=1  MassUnits=kg  MomentsOfInertia=[1 1 1]  MomentsOfInertiaUnits=kg*m^2  GraphicOpacity=1.0  ProductsOfInertia=[0 0 0]  ProductsOfInertiaUnits=kg*m^2  RevolutionCrossSection=[0.5 0.001; 0.5 -0.001; 0.75 -0.001; 0.75 0.001]*0.5  RevolutionCrossSectionUnits=m  RevolutionAngle=180  RevolutionAngleUnits=deg  RevolutionExtent=Full  GraphicShininess=75  GraphicSpecularColor=[0.5 0.5 0.5 1.0]  GraphicVisPropType=SimpleVisualProperties
  Target Outer Ring : sm_lib/Body Elements/Revolved Solid  Commented=on  GraphicAmbientColor=[0.15 0.15 0.15 1.0]  BasedOnType=Density  CenterOfMass=[0 0 0]  CenterOfMassUnits=m  GraphicDiffuseColor=[0.2 0.4 1.0]  ExportConvexHullGeometry=off  Density=1000  DensityUnits=kg/m^3  DoExposeReferenceFrame=on  GraphicEmissiveColor=[0.0 0.0 0.0 1.0]  ExportEntireGeometry=off  SerializedFrames=<Frames/>  MarkerShape=Sphere  MarkerSize=10  GraphicType=FromGeometry  InertiaType=CalculateFromGeometry  Mass=1  MassUnits=kg  MomentsOfInertia=[1 1 1]  MomentsOfInertiaUnits=kg*m^2  GraphicOpacity=1.0  ProductsOfInertia=[0 0 0]  ProductsOfInertiaUnits=kg*m^2  RevolutionCrossSection=[0.5 0.001; 0.5 -0.001; 0.75 -0.001; 0.75 0.001]  RevolutionCrossSectionUnits=m  RevolutionAngle=180  RevolutionAngleUnits=deg  RevolutionExtent=Full  GraphicShininess=75  GraphicSpecularColor=[0.5 0.5 0.5 1.0]  GraphicVisPropType=SimpleVisualProperties
  Conn1 : PMIOPort  Side=Left
  connections:
  Target Middle Ring/RConn1 -- Conn1/RConn1 -- Target Inner Ring/RConn1

== system simcape_real_time_V3/SIMCAPE/Subsystem5/Subsystem1 ==
  Target Inner Ring : sm_lib/Body Elements/Revolved Solid  GraphicAmbientColor=[0.15 0.15 0.15 1.0]  BasedOnType=Density  CenterOfMass=[0 0 0]  CenterOfMassUnits=m  GraphicDiffuseColor=[1.0 0.2 0.2]  ExportConvexHullGeometry=off  Density=1000  DensityUnits=kg/m^3  DoExposeReferenceFrame=on  GraphicEmissiveColor=[0.0 0.0 0.0 1.0]  ExportEntireGeometry=off  SerializedFrames=<Frames/>  MarkerShape=Sphere  MarkerSize=10  GraphicType=FromGeometry  InertiaType=CalculateFromGeometry  Mass=1  MassUnits=kg  MomentsOfInertia=[1 1 1]  MomentsOfInertiaUnits=kg*m^2  GraphicOpacity=1.0  ProductsOfInertia=[0 0 0]  ProductsOfInertiaUnits=kg*m^2  RevolutionCrossSection=[0.5 0.001; 0.5 -0.001; 0.75 -0.001; 0.75 0.001]*0.25  RevolutionCrossSectionUnits=m  RevolutionAngle=180  RevolutionAngleUnits=deg  RevolutionExtent=Full  GraphicShininess=75  GraphicSpecularColor=[0.5 0.5 0.5 1.0]  GraphicVisPropType=SimpleVisualProperties
  Target Middle Ring : sm_lib/Body Elements/Revolved Solid  GraphicAmbientColor=[0.15 0.15 0.15 1.0]  BasedOnType=Density  CenterOfMass=[0 0 0]  CenterOfMassUnits=m  GraphicDiffuseColor=[1.0 0.8 0.2]  ExportConvexHullGeometry=off  Density=1000  DensityUnits=kg/m^3  DoExposeReferenceFrame=on  GraphicEmissiveColor=[0.0 0.0 0.0 1.0]  ExportEntireGeometry=off  SerializedFrames=<Frames/>  MarkerShape=Sphere  MarkerSize=10  GraphicType=FromGeometry  InertiaType=CalculateFromGeometry  Mass=1  MassUnits=kg  MomentsOfInertia=[1 1 1]  MomentsOfInertiaUnits=kg*m^2  GraphicOpacity=1.0  ProductsOfInertia=[0 0 0]  ProductsOfInertiaUnits=kg*m^2  RevolutionCrossSection=[0.5 0.001; 0.5 -0.001; 0.75 -0.001; 0.75 0.001]*0.5  RevolutionCrossSectionUnits=m  RevolutionAngle=180  RevolutionAngleUnits=deg  RevolutionExtent=Full  GraphicShininess=75  GraphicSpecularColor=[0.5 0.5 0.5 1.0]  GraphicVisPropType=SimpleVisualProperties
  Target Outer Ring : sm_lib/Body Elements/Revolved Solid  Commented=on  GraphicAmbientColor=[0.15 0.15 0.15 1.0]  BasedOnType=Density  CenterOfMass=[0 0 0]  CenterOfMassUnits=m  GraphicDiffuseColor=[0.2 0.4 1.0]  ExportConvexHullGeometry=off  Density=1000  DensityUnits=kg/m^3  DoExposeReferenceFrame=on  GraphicEmissiveColor=[0.0 0.0 0.0 1.0]  ExportEntireGeometry=off  SerializedFrames=<Frames/>  MarkerShape=Sphere  MarkerSize=10  GraphicType=FromGeometry  InertiaType=CalculateFromGeometry  Mass=1  MassUnits=kg  MomentsOfInertia=[1 1 1]  MomentsOfInertiaUnits=kg*m^2  GraphicOpacity=1.0  ProductsOfInertia=[0 0 0]  ProductsOfInertiaUnits=kg*m^2  RevolutionCrossSection=[0.5 0.001; 0.5 -0.001; 0.75 -0.001; 0.75 0.001]  RevolutionCrossSectionUnits=m  RevolutionAngle=180  RevolutionAngleUnits=deg  RevolutionExtent=Full  GraphicShininess=75  GraphicSpecularColor=[0.5 0.5 0.5 1.0]  GraphicVisPropType=SimpleVisualProperties
  Conn1 : PMIOPort  Side=Left
  connections:
  Conn1/RConn1 -- Target Middle Ring/RConn1 -- Target Inner Ring/RConn1

== system simcape_real_time_V3/SIMCAPE/Subsystem5/Subsystem2 ==
  Target Inner Ring : sm_lib/Body Elements/Revolved Solid  GraphicAmbientColor=[0.15 0.15 0.15 1.0]  BasedOnType=Density  CenterOfMass=[0 0 0]  CenterOfMassUnits=m  GraphicDiffuseColor=[1.0 0.2 0.2]  ExportConvexHullGeometry=off  Density=1000  DensityUnits=kg/m^3  DoExposeReferenceFrame=on  GraphicEmissiveColor=[0.0 0.0 0.0 1.0]  ExportEntireGeometry=off  SerializedFrames=<Frames/>  MarkerShape=Sphere  MarkerSize=10  GraphicType=FromGeometry  InertiaType=CalculateFromGeometry  Mass=1  MassUnits=kg  MomentsOfInertia=[1 1 1]  MomentsOfInertiaUnits=kg*m^2  GraphicOpacity=1.0  ProductsOfInertia=[0 0 0]  ProductsOfInertiaUnits=kg*m^2  RevolutionCrossSection=[0.5 0.001; 0.5 -0.001; 0.75 -0.001; 0.75 0.001]*0.25  RevolutionCrossSectionUnits=m  RevolutionAngle=180  RevolutionAngleUnits=deg  RevolutionExtent=Full  GraphicShininess=75  GraphicSpecularColor=[0.5 0.5 0.5 1.0]  GraphicVisPropType=SimpleVisualProperties
  Target Middle Ring : sm_lib/Body Elements/Revolved Solid  GraphicAmbientColor=[0.15 0.15 0.15 1.0]  BasedOnType=Density  CenterOfMass=[0 0 0]  CenterOfMassUnits=m  GraphicDiffuseColor=[1.0 0.8 0.2]  ExportConvexHullGeometry=off  Density=1000  DensityUnits=kg/m^3  DoExposeReferenceFrame=on  GraphicEmissiveColor=[0.0 0.0 0.0 1.0]  ExportEntireGeometry=off  SerializedFrames=<Frames/>  MarkerShape=Sphere  MarkerSize=10  GraphicType=FromGeometry  InertiaType=CalculateFromGeometry  Mass=1  MassUnits=kg  MomentsOfInertia=[1 1 1]  MomentsOfInertiaUnits=kg*m^2  GraphicOpacity=1.0  ProductsOfInertia=[0 0 0]  ProductsOfInertiaUnits=kg*m^2  RevolutionCrossSection=[0.5 0.001; 0.5 -0.001; 0.75 -0.001; 0.75 0.001]*0.5  RevolutionCrossSectionUnits=m  RevolutionAngle=180  RevolutionAngleUnits=deg  RevolutionExtent=Full  GraphicShininess=75  GraphicSpecularColor=[0.5 0.5 0.5 1.0]  GraphicVisPropType=SimpleVisualProperties
  Target Outer Ring : sm_lib/Body Elements/Revolved Solid  Commented=on  GraphicAmbientColor=[0.15 0.15 0.15 1.0]  BasedOnType=Density  CenterOfMass=[0 0 0]  CenterOfMassUnits=m  GraphicDiffuseColor=[0.2 0.4 1.0]  ExportConvexHullGeometry=off  Density=1000  DensityUnits=kg/m^3  DoExposeReferenceFrame=on  GraphicEmissiveColor=[0.0 0.0 0.0 1.0]  ExportEntireGeometry=off  SerializedFrames=<Frames/>  MarkerShape=Sphere  MarkerSize=10  GraphicType=FromGeometry  InertiaType=CalculateFromGeometry  Mass=1  MassUnits=kg  MomentsOfInertia=[1 1 1]  MomentsOfInertiaUnits=kg*m^2  GraphicOpacity=1.0  ProductsOfInertia=[0 0 0]  ProductsOfInertiaUnits=kg*m^2  RevolutionCrossSection=[0.5 0.001; 0.5 -0.001; 0.75 -0.001; 0.75 0.001]  RevolutionCrossSectionUnits=m  RevolutionAngle=180  RevolutionAngleUnits=deg  RevolutionExtent=Full  GraphicShininess=75  GraphicSpecularColor=[0.5 0.5 0.5 1.0]  GraphicVisPropType=SimpleVisualProperties
  Conn1 : PMIOPort  Side=Left
  connections:
  Conn1/RConn1 -- Target Middle Ring/RConn1 -- Target Inner Ring/RConn1

== system simcape_real_time_V3/Subsystem/Quỹ đạo bậc 5/Subsystem ==
  Trigger : TriggerPort  VariantControl=Variant  PortDimensions=1
  Add : Sum
  Constant : Constant  OutDataTypeStr=double
  Data Store Read : DataStoreRead  DataStoreName=N_wp  DataStoreElements=N_wp  IndexOptions=Index vector (dialog)  Indices=1  OutputSizes=1
  Data Store Write : DataStoreWrite  DataStoreName=N_wp  DataStoreElements=N_wp  IndexOptions=Index vector (dialog)  Indices=1  OutputSizes=1
  Display : Display
  wires:
  Constant/1 -> Add/2
  Data Store Read/1 -> Add/1
  Add/1 -> Display/1, Data Store Write/1

== matlab function simcape_real_time_V3/MATLAB Function2 ==
  data: T1 input; D1 output; T2 input; T3 input; T4 input; D2 output; D3 output; D4 output
function [D1,D2,D3,D4]= fcn(T1,T2,T3,T4)
D1=(T1/11.5)*1000+1000;
D2=(T2/11.5)*1000+1000;
D3=(T3/11.5)*1000+1000;
D4=(T4/11.5)*1000+1000;

end

== matlab function simcape_real_time_V3/Subsystem4/Subsystem3/MATLAB Function1 ==
  data: Ux input; pitch_SP output; Uy input; yaw input; roll_SP input
function pitch_SP = fcn(Ux,Uy,yaw,roll_SP)

pitch_SP=(cos(yaw)*Ux+sin(yaw)*Uy)/cos(roll_SP);

end

== matlab function simcape_real_time_V3/Subsystem1/Quỹ đạo trục z/MATLAB Function10 ==
  data: q0 input; X output; qf input; v_qd input; V output; A output
function [X,V,A]= fcn(q0,qf,v_qd)
persistent t  a0 a1 a2 a3 a4 a5 

ts=0.002; %% thời gian lấy mẫu 

tf   = qf/v_qd; %% thời gian hoàn thành quãng đường

%% Quy hoạch quỹ đạo đa thức bậc 5

v0=0; % vận tốc nam đầu
ao=0; % gia tốc ban đầu

vf=0;   % vận tốc điểm cuối
af=0;   % gia tốc điểm cuối

a0 = q0;
a1 = v0;
a2 = ao/2;
a3 = -(20*q0 - 20*qf + 12*v0*tf + 8*vf*tf + 3*ao*tf^2 - af*tf^2)/(2*tf^3);
a4 = (30*q0 - 30*qf + 16*v0*tf + 14*vf*tf + 3*ao*tf^2 - 2*af*tf^2)/(2*tf^4);
a5 = -(12*q0 - 12*qf + 6*v0*tf + 6*vf*tf + ao*tf^2 - af*tf^2)/(2*tf^5);
          

if isempty(t)    
    t = 0;
end
%% thời gian ban đầu
    t = t + ts;
%     t_out = t;
 %% Check điều kiện dừng
if(t>tf)
    t=tf;
end

%% công thức tổng quát quỹ đạo bậc 5 vị trí theo thời gian t
X= a0 + a1*t + a2*t^2 + a3*t^3 + a4*t^4 + a5*t^5;
%% công thức tổng quát quỹ đạo bậc 5 vị trí theo thời gian t
V= a1 + 2*a2*t + 3*a3*t^2 + 4*a4*t^3 + 5*a5*t^4;
%% công thức tổng quát quỹ đạo bậc 5 vị trí theo thời gian t
A=  2*a2 + 6*a3*t + 12*a4*t^2 + 20*a5*t^3;
if(qf==0)
  X=0;
  V=0;
  A=0;
 end
end

== matlab function simcape_real_time_V3/Subsystem1/Quỹ đạo trục x/MATLAB Function10 ==
  data: q0 input; X output; qf input; v_qd input; V output; A output
function [X,V,A]= fcn(q0,qf,v_qd)
persistent t  a0 a1 a2 a3 a4 a5 

ts=0.002; %% thời gian lấy mẫu 

tf   = qf/v_qd; %% thời gian hoàn thành quãng đường

%% Quy hoạch quỹ đạo đa thức bậc 5

v0=0; % vận tốc nam đầu
ao=0; % gia tốc ban đầu

vf=0;   % vận tốc điểm cuối
af=0;   % gia tốc điểm cuối

a0 = q0;
a1 = v0;
a2 = ao/2;
a3 = -(20*q0 - 20*qf + 12*v0*tf + 8*vf*tf + 3*ao*tf^2 - af*tf^2)/(2*tf^3);
a4 = (30*q0 - 30*qf + 16*v0*tf + 14*vf*tf + 3*ao*tf^2 - 2*af*tf^2)/(2*tf^4);
a5 = -(12*q0 - 12*qf + 6*v0*tf + 6*vf*tf + ao*tf^2 - af*tf^2)/(2*tf^5);
          

if isempty(t)    
    t = 0;
end
%% thời gian ban đầu
    t = t + ts;
%     t_out = t;
 %% Check điều kiện dừng
if(t>tf)
    t=tf;
end

%% công thức tổng quát quỹ đạo bậc 5 vị trí theo thời gian t
X= a0 + a1*t + a2*t^2 + a3*t^3 + a4*t^4 + a5*t^5;
%% công thức tổng quát quỹ đạo bậc 5 vị trí theo thời gian t
V= a1 + 2*a2*t + 3*a3*t^2 + 4*a4*t^3 + 5*a5*t^4;
%% công thức tổng quát quỹ đạo bậc 5 vị trí theo thời gian t
A=  2*a2 + 6*a3*t + 12*a4*t^2 + 20*a5*t^3;
if(qf==0)
  X=0;
  V=0;
  A=0;
 end
end

== matlab function simcape_real_time_V3/Subsystem1/Quỹ đạo trục y/MATLAB Function10 ==
  data: q0 input; X output; qf input; v_qd input; V output; A output
function [X,V,A]= fcn(q0,qf,v_qd)
persistent t  a0 a1 a2 a3 a4 a5 

ts=0.002; %% thời gian lấy mẫu 

tf   = qf/v_qd; %% thời gian hoàn thành quãng đường


%% Quy hoạch quỹ đạo đa thức bậc 5

v0=0; % vận tốc nam đầu
ao=0; % gia tốc ban đầu

vf=0;   % vận tốc điểm cuối
af=0;   % gia tốc điểm cuối

a0 = q0;
a1 = v0;
a2 = ao/2;
a3 = -(20*q0 - 20*qf + 12*v0*tf + 8*vf*tf + 3*ao*tf^2 - af*tf^2)/(2*tf^3);
a4 = (30*q0 - 30*qf + 16*v0*tf + 14*vf*tf + 3*ao*tf^2 - 2*af*tf^2)/(2*tf^4);
a5 = -(12*q0 - 12*qf + 6*v0*tf + 6*vf*tf + ao*tf^2 - af*tf^2)/(2*tf^5);
          

if isempty(t)    
    t = 0;
end
%% thời gian ban đầu
    t = t + ts;
%     t_out = t;
 %% Check điều kiện dừng
if(t>tf)
    t=tf;
end

%% công thức tổng quát quỹ đạo bậc 5 vị trí theo thời gian t
X= a0 + a1*t + a2*t^2 + a3*t^3 + a4*t^4 + a5*t^5;
%% công thức tổng quát quỹ đạo bậc 5 vị trí theo thời gian t
V= a1 + 2*a2*t + 3*a3*t^2 + 4*a4*t^3 + 5*a5*t^4;
%% công thức tổng quát quỹ đạo bậc 5 vị trí theo thời gian t
A=  2*a2 + 6*a3*t + 12*a4*t^2 + 20*a5*t^3;

if(qf==0)
  X=0;
  V=0;
  A=0;
 end
end

== matlab function simcape_real_time_V3/G00(xyzv)/MATLAB Function1 ==
  data: xyzv_in input; xyzv_out output
function xyzv_out = fcn(xyzv_in)
        
        x_out = xyzv_in(1);
        y_out = xyzv_in(2);
        z_out = xyzv_in(3);
        v_out = xyzv_in(4);
        
        xyzv_out  = [x_out ; y_out ; z_out ; v_out ];
end

== matlab function simcape_real_time_V3/Subsystem4/Subsystem/MATLAB Function7 ==
  settings: updateMethod=DISCRETE
  data: roll input; pitch input; z_2dot_SP input; z_dot_SP input; z_SP input; a1 input; a0 input; K input; z input; z_dot input; U1 output; ez output; ez_dot output
function [U1,ez,ez_dot]= fcn(roll,pitch,z_2dot_SP,z_dot_SP,z_SP,a1,a0,K,z,z_dot)  
    %% khai báo biến hệ thống
    g=9.81;
    m=1.7;
    %% phương trình trạng thái
    % z_2dot=((U1*cos(pitch)*cos(roll))/m) - g;
    %% Chọn phương trình mặt trượt có dạng
    ez=z_SP-z;
    ez_dot=z_dot_SP-z_dot;
    Sz=a1*(z_dot_SP-z_dot)+a0*(z_SP-z);
    %% Chọn tiêu chí tốc độ hội tụ, trong đó K là hệ số dương Nếu K càng lớn thì độ hội tụ về 0 càng giảm
    VSz_dot=-K*sign(Sz);
    %% Thiết kế tín hiệu điều khiển Ux Uy
    U1=(m/(cos(roll)*cos(pitch)))*(z_2dot_SP+K*sign(Sz)*abs(Sz)+g+a0*(z_dot_SP-z_dot));
end

== matlab function simcape_real_time_V3/Subsystem4/Subsystem1/MATLAB Function7 ==
  data: U1 input; y_2dot_SP input; y_dot_SP input; y_SP input; a1 input; a0 input; Uy output; K input; y input; y_dot input; ey output; ey_dot output
function [Uy,ey,ey_dot]= fcn(U1,y_2dot_SP,y_dot_SP,y_SP,a1,a0,K,y,y_dot) 

%% khai báo biến hệ thống
m=1.7;

%% phương trình trạng thái

% y_2dot=-(U1*cos(yaw)*sin(roll) - cos(roll)*sin(pitch)*sin(yaw))/m;

%% Chọn phương trình mặt trượt có dạng
ey=y_SP-y;
ey_dot=y_dot_SP-y_dot;
Sy=a1*(ey_dot)+a0*(ey);

%% Chọn tiêu chí tốc độ hội tụ, trong đó K là hệ số dương Nếu K càng lớn thì độ hội tụ về 0 càng giảm

VSy=-K*sign(Sy);

%% Thiết kế tín hiệu điều khiển Ux Uy

Uy=(m/U1)*(y_2dot_SP+a0*(y_dot_SP-y_dot)+K*sign(Sy)*abs(Sy));

end

== matlab function simcape_real_time_V3/Subsystem4/Subsystem1/MATLAB Function9 ==
  data: U1 input; x_2dot_SP input; x_dot_SP input; x_SP input; a1 input; a0 input; K input; Ux output; x input; x_dot input; ex_dot output; ex output
function [Ux,ex_dot,ex]= fcn(U1,x_2dot_SP,x_dot_SP,x_SP,a1,a0,K,x,x_dot) 

%% khai báo biến hệ thống

m=1.7;

%% phương trình trạng thái

% x_2dot=(U1*sin(roll)*sin(yaw) + cos(roll)*cos(yaw)*sin(pitch))/m;

%% Chọn phương trình mặt trượt có dạng
ex=x_SP-x;
ex_dot=x_dot_SP-x_dot;
Sx=a1*(ex_dot)+a0*(ex);

%% Chọn tiêu chí tốc độ hội tụ, trong đó K là hệ số dương Nếu K càng lớn thì độ hội tụ về 0 càng giảm

VSx=-K*sign(Sx);

%% Thiết kế tín hiệu điều khiển Ux Uy

Ux=(m/U1)*(x_2dot_SP+a0*(x_dot_SP-x_dot)+K*sign(Sx)*abs(Sx));

end

== matlab function simcape_real_time_V3/Subsystem4/Subsystem3/MATLAB Function8 ==
  data: Ux input; roll_SP output; Uy input; yaw input
function roll_SP = fcn(Ux,Uy,yaw)

roll_SP=(sin(yaw)*Ux)-(cos(yaw)*Uy);

end

== matlab function simcape_real_time_V3/Subsystem/Quỹ đạo bậc 5/MATLAB Function13 ==
  data: V_AB_t output; xyzv input; PhanTram_S output; Px output; Py output; Pz output; x_a_save output; y_a_save output; z_a_save output; t_save output; x_a_pre input; y_a_pre input; z_a_pre input; t input
function [V_AB_t,PhanTram_S,Px,Py,Pz,x_a_save,y_a_save,z_a_save,t_save]= fcn(xyzv,x_a_pre,y_a_pre,z_a_pre,t)
    x_b=xyzv(1);
    y_b=xyzv(2);
    z_b=xyzv(3);
    v_tb=xyzv(4);
    AB = sqrt((x_b-x_a_pre)^2+(y_b-y_a_pre)^2+(z_b-z_a_pre)^2);
    if(v_tb>0)
        tf = AB/v_tb;
    else
        tf=0;
    end
    ts = 0.002; 
    %% Nội suy Phần tram quãng đường liên tục theo thời gian theo phương pháp quy hoạch quỹ đạo bậc 5
    q0 = 0;
    qf = AB;

    a_0 = q0;
    a_1 = 0;
    a_2 = 0;
    a_3 = ((20*qf)/(2*tf*tf*tf));
    a_4 = ((-30*qf)/(2*tf*tf*tf*tf));
    a_5 = ((12*qf)/(2*tf*tf*tf*tf*tf));
    t=t+ts;
    if(t<tf)
        t_save=t;
        temp=0;
    elseif(t==tf)
        t_save=0;
        temp=1;
    elseif(t>tf)
        t = tf;
        t_save=0;
        temp=1;
    else
        t_save = 0;
        temp = 1;
        t = 0;
    end

    if(AB==0)||(temp==1)
        S_t = AB;
        V_AB_t = 0;
    else
        S_t = a_0+ (a_1*t) + (a_2*t*t) + (a_3*t*t*t) + (a_4*t*t*t*t) + (a_5*t*t*t*t*t);
        V_AB_t = a_1 + (2*a_2*t) + (3*a_3*t*t) + (4*a_4*t*t*t) + (5*a_5*t*t*t*t);
    end
    %%%
    PhanTram_S = (S_t*100)/AB;
    %% Nội suy tọa độ theo công thức hình học.
    if(temp==1)
        Px=x_b;
        Py=y_b;
        Pz=z_b;
        x_a_save=x_b;
        y_a_save=y_b;
        z_a_save=z_b;
    else
        x_a_save=x_a_pre;
        y_a_save=y_a_pre;
        z_a_save=z_a_pre;
        Px = x_a_pre + S_t*(x_b-x_a_pre)/AB;
        Py = y_a_pre + S_t*(y_b-y_a_pre)/AB;
        Pz = z_a_pre + S_t*(z_b-z_a_pre)/AB;
    end
    % vx=(Px-Px_save)/ts;
    % vy=(Py-Py_save)/ts;
    % vz=(Pz-Pz_save)/ts;
    % v_tt=sqrt(vx*vx+vy*vy+vz*vz);
    % a_tt=(v_tt - v_tt_save)/ts;
    % Px_save=Px;
    % Py_save=Py;
    % Pz_save=Pz;
    % v_tt_save=v_tt;
     
end

== matlab function simcape_real_time_V3/call1 ==
  data: N_wp input
function fcn(N_wp)
    switch(N_wp)  
        case 1
        MoveL([0;0;100;20]);
        case 2
        MoveL([-300;0;100;50]);
        case 3
        MoveL([-300;-300;100;50]);
        case 4
        MoveL([-300;-300;150;50]);
%         case 5
%         MoveL([-300;0;150;50]);
%         case 6
%         MoveL([0;0;150;50]);
%         case 7
%         MoveL([0;0;0;50]); 
    end
end

== matlab function simcape_real_time_V3/Subsystem/Quỹ đạo bậc 5/MATLAB Function ==
  data: Px input; v_tt output; Py input; Pz input; Px_save input; Py_save input; Pz_save input; vx output; vy output; vz output
function [v_tt ,vx,vy,vz]= fcn(Px,Py,Pz,Px_save,Py_save,Pz_save)
  ts=0.002;
  vx=(Px-Px_save)/ts;
  vy=(Py-Py_save)/ts;
  vz=(Pz-Pz_save)/ts;
  v_tt=sqrt((vx*vx)+(vy*vy)+(vz*vz));
end

== matlab function simcape_real_time_V3/Subsystem/Quỹ đạo bậc 5/MATLAB Function1 ==
  data: vx input; ax output; vx_save input; vy input; vy_save input; vz input; vz_save input; ay output; az output
function [ax,ay,az]= fcn(vx,vx_save,vy,vy_save,vz,vz_save)
    ts=0.002;
    ax=(vx-vx_save)/ts;
    ay=(vy-vy_save)/ts;
    az=(vz-vz_save)/ts;
end

== matlab function simcape_real_time_V3/MATLAB Function1 ==
  data: D1 input; T1 output; D2 input; D3 input; D4 input; T2 output; T3 output; T4 output
function [T1,T2,T3,T4]= fcn(D1,D2,D3,D4)
T1=(D1-1000)/1000*11.5;
T2=(D2-1000)/1000*11.5;
T3=(D3-1000)/1000*11.5;
T4=(D4-1000)/1000*11.5;

end
